simulink model "casperdemo"  (Simulink 6.2)
settings: Solver=ode45  StartTime=0.0  StopTime=16384  RelTol=1e-3
libraries: xbsIndex_r3 x1645, casper_library x163, testbench_lib x15, xps_library x1
(part 1 of 12)
settings Model: LastModifiedBy=Glenn
settings DebuggingCC: SolverPrmCheckMsg=warning

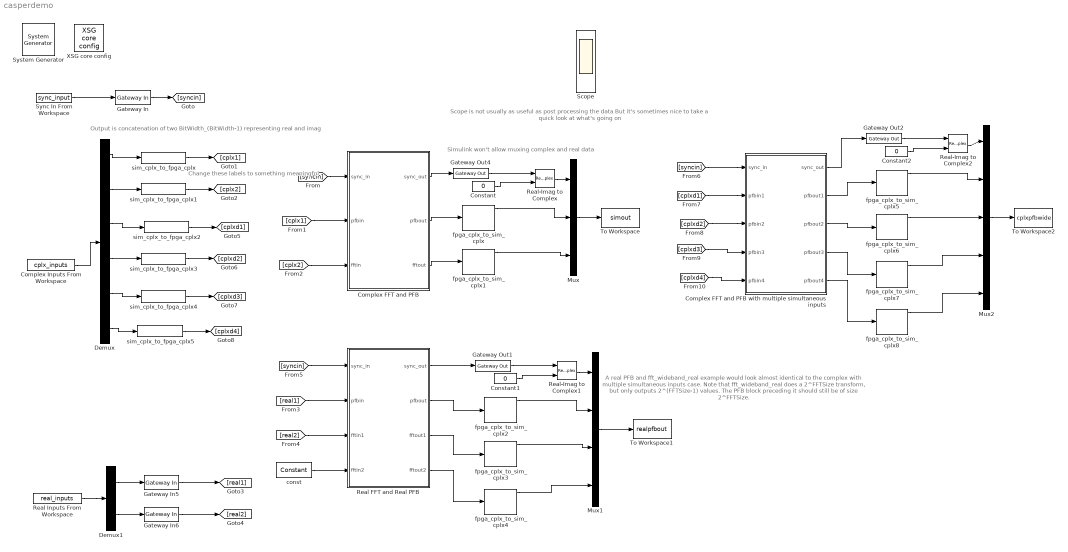
== system casperdemo ==
  note: Output is concatenation of two BitWidth_(BitWidth-1)
      | representing real and imag
  note: Change these labels to
      | something meaningful
  note: Simulink won't allow muxing
      | complex and real data
  note: Scope is not usually as useful as post processing the data
      | But it's sometimes nice to take a quick look at what's going on
  note: A real PFB and fft_wideband_real example would
      | look almost identical to the complex with multiple simultaneous
      | inputs case. Note that fft_wideband_real does a 2^FFTSize
      | transform, but only outputs 2^(FFTSize-1) values.
      | The PFB block preceding it should still be of size 2^FFTSize.
  " System Generator" : xbsIndex_r3/ System Generator  Tag=genX  xilinxfamily=Virtex2  part=xc2v1000  speed=-4  package=bg575  synthesis_tool=XST  directory=./netlist  testbench=off  simulink_period=1  sysclk_period=100  incr_netlist=off  trim_vbits=Everywhere in SubSystem  dbl_ovrd=According to Block Masks  core_generation=According to Block Masks  run_coregen=off  deprecated_control=off  eval_field=0
      settings: AttributesFormatString=System\nGenerator
  Complex FFT and PFB : Subsystem
  Complex FFT and PFB with multiple simultaneous inputs : Subsystem
  Complex Inputs From Workspace : FromWorkspace  VariableName=cplx_inputs  SampleTime=1  Interpolate=off  OutputAfterFinalValue=Setting to zero
  Constant : Constant  Value=0
  Constant1 : Constant  Value=0
  Constant2 : Constant  Value=0
  Demux : Demux  Outputs=6
  Demux1 : Demux  Outputs=2
  Gateway In : xbsIndex_r3/Gateway In  arith_type=Boolean  n_bits=8  bin_pt=6  quantization=Truncate  overflow=Wrap  period=1  timing_constraint=None  locs_specified=off  LOCs={}  needs_fixed_name=off  dbl_ovrd=off  show_param=off
      settings: xl_area=[0, 0, 0, 0, 0, 0, 0]
  Gateway In5 : xbsIndex_r3/Gateway In  arith_type="Signed  (2's comp)"  n_bits=8  bin_pt=7  quantization=Truncate  overflow=Wrap  period=1  timing_constraint=None  locs_specified=off  LOCs={}  needs_fixed_name=off  dbl_ovrd=off  show_param=off
      settings: xl_area=[0, 0, 0, 0, 0, 0, 0]
  Gateway In6 : xbsIndex_r3/Gateway In  arith_type="Signed  (2's comp)"  n_bits=18  bin_pt=17  quantization=Truncate  overflow=Wrap  period=1  timing_constraint=None  locs_specified=off  LOCs={}  needs_fixed_name=off  dbl_ovrd=off  show_param=off
      settings: xl_area=[0, 0, 0, 0, 0, 0, 0]
  Gateway Out1 : xbsIndex_r3/Gateway Out  output_type=Double  nbits=8  bin_pt=6  arith_type=Boolean  quantization=Truncate  overflow=Wrap  hdl_port=on  timing_constraint=None  locs_specified=off  LOCs={}  needs_fixed_name=off  show_param=off
      settings: xl_area=[0, 0, 0, 0, 0, 0, 0]
  Gateway Out2 : xbsIndex_r3/Gateway Out  output_type=Double  nbits=8  bin_pt=6  arith_type=Boolean  quantization=Truncate  overflow=Wrap  hdl_port=on  timing_constraint=None  locs_specified=off  LOCs={}  needs_fixed_name=off  show_param=off
      settings: xl_area=[0, 0, 0, 0, 0, 0, 0]
  Gateway Out4 : xbsIndex_r3/Gateway Out  output_type=Double  nbits=8  bin_pt=6  arith_type=Boolean  quantization=Truncate  overflow=Wrap  hdl_port=on  timing_constraint=None  locs_specified=off  LOCs={}  needs_fixed_name=off  show_param=off
      settings: xl_area=[0, 0, 0, 0, 0, 0, 0]
  Mux : Mux  Inputs=3
  Mux1 : Mux
  Mux2 : Mux  Inputs=5
  Real FFT and Real PFB : Subsystem
  Real Inputs From Workspace : FromWorkspace  VariableName=real_inputs  SampleTime=1  Interpolate=off  OutputAfterFinalValue=Setting to zero
  Real-Imag to Complex : RealImagToComplex
  Real-Imag to Complex1 : RealImagToComplex
  Real-Imag to Complex2 : RealImagToComplex
  Scope : Scope  NumInputPorts=4
      settings: YMin=-1~-0.5~-0.5~-1  YMax=1~0.5~0.5~1
  Sync In From Workspace : FromWorkspace  VariableName=sync_input  SampleTime=1  Interpolate=off  OutputAfterFinalValue=Setting to zero
  To Workspace : ToWorkspace  VariableName=simout  SampleTime=-1  SaveFormat=Structure
  To Workspace1 : ToWorkspace  VariableName=realpfbout  SampleTime=-1  SaveFormat=Structure
  To Workspace2 : ToWorkspace  VariableName=cplxpfbwide  SampleTime=-1  SaveFormat=Structure
  XSG core config : xps_library/XSG core config  Tag=xps:xsg  hw_sys=iBOB  ibob_linux=off  clk_src=sys_clk  gpio_clk_io_group=iBOB:sma  gpio_clk_bit_index=0  clk_rate=100  sample_period=1  synthesis_tool=XST  mpc_type=powerpc405
  const : xbsIndex_r3/Constant  const=.1  equ=P=C  arith_type="Signed  (2's comp)"  n_bits=18  bin_pt=17  opselect=C  inp2=PCIN>>17  opr=+  inp1=P  carry=CIN  iostate=0  explicit_period=on  period=1  dbl_ovrd=off
  fpga_cplx_to_sim_cplx{,1..8} (9 alike) : testbench_lib/fpga_cplx_to_sim_cplx  width=18
      settings: AttributesFormatString=18_17 bit
  sim_cplx_to_fpga_cplx{,2..5} (5 alike) : testbench_lib/sim_cplx_to_fpga_cplx  width=8
      settings: AttributesFormatString=8_7 bit
  sim_cplx_to_fpga_cplx1 : testbench_lib/sim_cplx_to_fpga_cplx  width=18
      settings: AttributesFormatString=18_17 bit
  wires:
  Sync In From Workspace/1 -> Gateway In/1
  Complex Inputs From Workspace/1 -> Demux/1
  Demux/1 -> sim_cplx_to_fpga_cplx/1
  Demux/2 -> sim_cplx_to_fpga_cplx1/1
  Real Inputs From Workspace/1 -> Demux1/1
  Demux1/1 -> Gateway In5/1
  Demux1/2 -> Gateway In6/1
  Gateway In/1 -> [syncin]
  sim_cplx_to_fpga_cplx/1 -> [cplx1]
  sim_cplx_to_fpga_cplx1/1 -> [cplx2]
  Gateway In5/1 -> [real1]
  Gateway In6/1 -> [real2]
  [syncin] -> Complex FFT and PFB/1(sync_in)
  [cplx1] -> Complex FFT and PFB/2(pfbin)
  Complex FFT and PFB/1(sync_out) -> Gateway Out4/1
  Complex FFT and PFB/2(pfbout) -> fpga_cplx_to_sim_cplx/1
  Complex FFT and PFB/3(fftout) -> fpga_cplx_to_sim_cplx1/1
  Gateway Out4/1 -> Real-Imag to Complex/1
  Constant/1 -> Real-Imag to Complex/2
  Real-Imag to Complex/1 -> Mux/1
  fpga_cplx_to_sim_cplx/1 -> Mux/2
  fpga_cplx_to_sim_cplx1/1 -> Mux/3
  Mux/1 -> To Workspace/1
  [cplx2] -> Complex FFT and PFB/3(fftin)
  [syncin] -> Real FFT and Real PFB/1(sync_in)
  [real1] -> Real FFT and Real PFB/2(pfbin)
  [real2] -> Real FFT and Real PFB/3(fftin1)
  const/1 -> Real FFT and Real PFB/4(fftin2)
  Gateway Out1/1 -> Real-Imag to Complex1/1
  Constant1/1 -> Real-Imag to Complex1/2
  Real-Imag to Complex1/1 -> Mux1/1
  fpga_cplx_to_sim_cplx2/1 -> Mux1/2
  fpga_cplx_to_sim_cplx3/1 -> Mux1/3
  Mux1/1 -> To Workspace1/1
  Real FFT and Real PFB/1(sync_out) -> Gateway Out1/1
  Real FFT and Real PFB/2(pfbout) -> fpga_cplx_to_sim_cplx2/1
  Real FFT and Real PFB/3(fftout1) -> fpga_cplx_to_sim_cplx3/1
  Real FFT and Real PFB/4(fftout2) -> fpga_cplx_to_sim_cplx4/1
  fpga_cplx_to_sim_cplx4/1 -> Mux1/4
  Demux/3 -> sim_cplx_to_fpga_cplx2/1
  Demux/4 -> sim_cplx_to_fpga_cplx3/1
  Demux/5 -> sim_cplx_to_fpga_cplx4/1
  Demux/6 -> sim_cplx_to_fpga_cplx5/1
  sim_cplx_to_fpga_cplx2/1 -> [cplxd1]
  sim_cplx_to_fpga_cplx3/1 -> [cplxd2]
  sim_cplx_to_fpga_cplx4/1 -> [cplxd3]
  sim_cplx_to_fpga_cplx5/1 -> [cplxd4]
  [syncin] -> Complex FFT and PFB with multiple simultaneous inputs/1(sync_in)
  [cplxd1] -> Complex FFT and PFB with multiple simultaneous inputs/2(pfbin1)
  [cplxd2] -> Complex FFT and PFB with multiple simultaneous inputs/3(pfbin2)
  [cplxd3] -> Complex FFT and PFB with multiple simultaneous inputs/4(pfbin3)
  [cplxd4] -> Complex FFT and PFB with multiple simultaneous inputs/5(pfbin4)
  Gateway Out2/1 -> Real-Imag to Complex2/1
  Constant2/1 -> Real-Imag to Complex2/2
  Real-Imag to Complex2/1 -> Mux2/1
  fpga_cplx_to_sim_cplx5/1 -> Mux2/2
  fpga_cplx_to_sim_cplx6/1 -> Mux2/3
  Mux2/1 -> To Workspace2/1
  fpga_cplx_to_sim_cplx7/1 -> Mux2/4
  fpga_cplx_to_sim_cplx8/1 -> Mux2/5
  Complex FFT and PFB with multiple simultaneous inputs/1(sync_out) -> Gateway Out2/1
  Complex FFT and PFB with multiple simultaneous inputs/2(pfbout1) -> fpga_cplx_to_sim_cplx5/1
  Complex FFT and PFB with multiple simultaneous inputs/3(pfbout2) -> fpga_cplx_to_sim_cplx6/1
  Complex FFT and PFB with multiple simultaneous inputs/4(pfbout3) -> fpga_cplx_to_sim_cplx7/1
  Complex FFT and PFB with multiple simultaneous inputs/5(pfbout4) -> fpga_cplx_to_sim_cplx8/1

== system casperdemo/Complex FFT and PFB ==
  note: With "Number of Simultaneous Inputs" = 2^0,
      | each input represents an independant data stream
      | processed simultaneously by the biplex structure.
      | Each segment of the input time series
      |  of length 2^FFTSize is transformed and
      | output as 2^FFTSize frequency points.
  sync_in : Inport  Port=1  LatchInput=off
  pfbin : Inport  Port=2  LatchInput=off
  fftin : Inport  Port=3  LatchInput=off
  fft : Subsystem  AncestorBlock=casper_library/FFTs/fft  mask(fft){FFTSize=4, BitWidth=18, n_inputs=0, quantization=Truncate, overflow=Wrap, add_latency=2, mult_latency=3, bram_latency=2}
      mask prompts: FFTSize "Size of FFT: (2^?)"; BitWidth "Bit Width"; n_inputs "Number of Simultaneous Inputs: (2^?)"; quantization "Quantization Behavior"; overflow "Overflow Behavior"; add_latency "Add Latency"; mult_latency "Mult Latency"; bram_latency "BRAM Latency"
      mask init:
      | fft_init(gcb,...
      |     'FFTSize', FFTSize,...
      |     'BitWidth', BitWidth,...
      |     'n_inputs', n_inputs,...
      |     'quantization', quantization,...
      |     'overflow', overflow,...
      |     'add_latency', add_latency,...
      |     'mult_latency', mult_latency,...
      |     'bram_latency', bram_latency);
      settings: AttributesFormatString=FFTSize=4, n_inputs=0
      mask StyleString: edit,edit,edit,popup(Truncate|Round  (unbiased: +/- Inf)|Round  (unbiased: Even Values)),popup(Wrap|Saturate|Error),edit,edit,edit
  pfb_fir : Subsystem  AncestorBlock=casper_library/PFBs/pfb_fir  mask(pfb_fir){PFBSize=4, TotalTaps=4, WindowType=hamming, n_inputs=0, MakeBiplex=1, BitWidthIn=8, BitWidthOut=18, CoeffBitWidth=8, CoeffDistMem=1, add_latency=1, mult_latency=2, bram_latency=2, quantization=Truncate, fwidth=1}
      mask prompts: PFBSize "Size of PFB: (2^? pnts)"; TotalTaps "Total Number of Taps:"; WindowType "Windowing Function:"; n_inputs "Number of Simultaneous Inputs: (2^?)"; MakeBiplex "Make Biplex"; BitWidthIn "Input Bitwidth:"; BitWidthOut "Output Bitwidth:"; CoeffBitWidth "Coefficient Bitwidth:"; CoeffDistMem "Use Distributed Memory for Coeffs"; add_latency "Add Latency"; mult_latency "Mult Latency"; bram_latency "BRAM Latency"; quantization "Quantization Behavior"; fwidth "Bin Width Scaling (normal=1)"
      mask init:
      | pfb_fir_init(gcb, ...
      |     'PFBSize', PFBSize, ...
      |     'TotalTaps', TotalTaps, ...
      |     'WindowType', WindowType, ...
      |     'n_inputs', n_inputs, ...
      |     'MakeBiplex', MakeBiplex, ...
      |     'BitWidthIn', BitWidthIn, ...
      |     'BitWidthOut', BitWidthOut, ...
      |     'CoeffBitWidth', CoeffBitWidth, ...
      |     'CoeffDistMem', CoeffDistMem, ...
      |     'add_latency', add_latency, ...
      |     'mult_latency', mult_latency, ...
      |     'bram_latency', bram_latency, ...
      |     'quantization', quantization, ...
      |     'fwidth', fwidth);
      settings: AttributesFormatString=taps=4, add_latency=1
      mask StyleString: edit,edit,popup(bartlett|barthannwin|blackman|blackmanharris|bohamwin|chebwin|flattopwin|gausswin|hamming|hann|kaiser|nuttallwin|parzenwin|rectwin|tukeywin|triang),edit,edit,edit,edit,edit,edit,edit,edit,edit,popup(Truncate|Round  (unbiased: +/- Inf)|Round  (unbiased: Even Values)),edit
  shift : xbsIndex_r3/Constant  const=-1  equ=P=C  arith_type="Signed  (2's comp)"  n_bits=32  bin_pt=0  opselect=C  inp2=PCIN>>17  opr=+  inp1=P  carry=CIN  iostate=0  explicit_period=on  period=1  dbl_ovrd=off
  sync_out : Outport
  pfbout : Outport  Port=2
  fftout : Outport  Port=3
  wires:
  sync_in/1 -> pfb_fir/1(sync)
  fft/1(sync_out) -> sync_out/1
  shift/1 -> fft/2(shift)
  fft/2(out0) -> pfbout/1
  fft/3(out1) -> fftout/1
  pfb_fir/1(sync_out) -> fft/1(sync)
  pfb_fir/2(pol1_out1) -> fft/3(pol0)
  pfbin/1 -> pfb_fir/2(pol1_in1), pfb_fir/3(pol2_in1)
  fftin/1 -> fft/4(pol1)

== system casperdemo/Complex FFT and PFB with multiple simultaneous inputs ==
  note: With "Number of Simultaneous Inputs" = 2^2,
      | the four inputs represent successive time samples
      | of the overall timeseries. They should be thought of in
      | blocks, for example as (x0,x1,x2,x3) come in on one clock
      | then (x4,x5,x6,x7) on the next clock. The outputs come out in
      | the same fashion. Thus if FFTSize=5, with 4 inputs at a time,
      | we get a full spectrum every 32/4 = 8 clocks.
  note: This could be hooked to a set of four
      | real/imag to complex blocks, with
      | the real ports driven by the I ADC inputs
      | and the imag ports driven by the Q ADC inputs
  sync_in : Inport  Port=1  LatchInput=off
  pfbin1 : Inport  Port=2  LatchInput=off
  pfbin2 : Inport  Port=3  LatchInput=off
  pfbin3 : Inport  Port=4  LatchInput=off
  pfbin4 : Inport  Port=5  LatchInput=off
  fft : Subsystem  AncestorBlock=casper_library/FFTs/fft  mask(fft){FFTSize=5, BitWidth=18, n_inputs=2, quantization=Truncate, overflow=Wrap, add_latency=2, mult_latency=3, bram_latency=2}
      mask prompts: FFTSize "Size of FFT: (2^?)"; BitWidth "Bit Width"; n_inputs "Number of Simultaneous Inputs: (2^?)"; quantization "Quantization Behavior"; overflow "Overflow Behavior"; add_latency "Add Latency"; mult_latency "Mult Latency"; bram_latency "BRAM Latency"
      mask init: same as casperdemo/Complex FFT and PFB/fft
      settings: AttributesFormatString=FFTSize=5, n_inputs=2
      mask StyleString: edit,edit,edit,popup(Truncate|Round  (unbiased: +/- Inf)|Round  (unbiased: Even Values)),popup(Wrap|Saturate|Error),edit,edit,edit
  pfb_fir : Subsystem  AncestorBlock=casper_library/PFBs/pfb_fir  mask(pfb_fir){PFBSize=5, TotalTaps=4, WindowType=hamming, n_inputs=2, MakeBiplex=0, BitWidthIn=8, BitWidthOut=18, CoeffBitWidth=8, CoeffDistMem=1, add_latency=1, mult_latency=2, bram_latency=2, quantization=Truncate, fwidth=1}
      mask prompts: PFBSize "Size of PFB: (2^? pnts)"; TotalTaps "Total Number of Taps:"; WindowType "Windowing Function:"; n_inputs "Number of Simultaneous Inputs: (2^?)"; MakeBiplex "Make Biplex"; BitWidthIn "Input Bitwidth:"; BitWidthOut "Output Bitwidth:"; CoeffBitWidth "Coefficient Bitwidth:"; CoeffDistMem "Use Distributed Memory for Coeffs"; add_latency "Add Latency"; mult_latency "Mult Latency"; bram_latency "BRAM Latency"; quantization "Quantization Behavior"; fwidth "Bin Width Scaling (normal=1)"
      mask init: same as casperdemo/Complex FFT and PFB/pfb_fir
      settings: AttributesFormatString=taps=4, add_latency=1
      mask StyleString: edit,edit,popup(bartlett|barthannwin|blackman|blackmanharris|bohamwin|chebwin|flattopwin|gausswin|hamming|hann|kaiser|nuttallwin|parzenwin|rectwin|tukeywin|triang),edit,edit,edit,edit,edit,edit,edit,edit,edit,popup(Truncate|Round  (unbiased: +/- Inf)|Round  (unbiased: Even Values)),edit
  shift : xbsIndex_r3/Constant  const=-1  equ=P=C  arith_type="Signed  (2's comp)"  n_bits=32  bin_pt=0  opselect=C  inp2=PCIN>>17  opr=+  inp1=P  carry=CIN  iostate=0  explicit_period=on  period=1  dbl_ovrd=off
  sync_out : Outport
  pfbout1 : Outport  Port=2
  pfbout2 : Outport  Port=3
  pfbout3 : Outport  Port=4
  pfbout4 : Outport  Port=5
  wires:
  pfbin1/1 -> pfb_fir/2(pol1_in1)
  pfb_fir/1(sync_out) -> fft/1(sync)
  shift/1 -> fft/2(shift)
  fft/1(sync_out) -> sync_out/1
  sync_in/1 -> pfb_fir/1(sync)
  pfb_fir/2(pol1_out1) -> fft/3(in0)
  pfb_fir/3(pol1_out2) -> fft/4(in1)
  pfb_fir/4(pol1_out3) -> fft/5(in2)
  pfb_fir/5(pol1_out4) -> fft/6(in3)
  pfbin2/1 -> pfb_fir/3(pol1_in2)
  pfbin3/1 -> pfb_fir/4(pol1_in3)
  pfbin4/1 -> pfb_fir/5(pol1_in4)
  fft/2(out0) -> pfbout1/1
  fft/3(out1) -> pfbout2/1
  fft/4(out2) -> pfbout3/1
  fft/5(out3) -> pfbout4/1

== system casperdemo/Real FFT and Real PFB ==
  note: Each input represents an independant data stream
      | Each segment of the input time series
      |  of length 2^FFTSize is transformed and
      | output as 2^FFTSize frequency points.
      | Negative frequencies included.
  sync_in : Inport  Port=1  LatchInput=off
  pfbin : Inport  Port=2  LatchInput=off
  fftin1 : Inport  Port=3  LatchInput=off
  fftin2 : Inport  Port=4  LatchInput=off
  fft_biplex_real_4x : Subsystem  AncestorBlock=casper_library/FFTs/fft_biplex_real_4x  mask(fft_biplex_real_4x){FFTSize=4, BitWidth=18, quantization=Truncate, overflow=Wrap, add_latency=2, mult_latency=3, bram_latency=2}
      mask prompts: FFTSize "Size of FFT: (2^? pnts)"; BitWidth "Bitwidth: (Max Efficiency at 18 bits)"; quantization "Quantization Behavior"; overflow "Overflow Behavior"; add_latency "Add Latency"; mult_latency "Mult Latency"; bram_latency "BRAM Latency"
      mask init:
      | fft_biplex_real_4x_init(gcb,...
      |     'FFTSize', FFTSize,...
      |     'BitWidth', BitWidth,...
      |     'quantization', quantization,...
      |     'overflow', overflow,...
      |     'add_latency', add_latency,...
      |     'mult_latency', mult_latency,...
      |     'bram_latency', bram_latency);
      settings: AttributesFormatString=FFTSize=4, BitWidth=18
      mask StyleString: edit,edit,popup(Truncate|Round  (unbiased: +/- Inf)|Round  (unbiased: Even Values)),popup(Wrap|Saturate|Error),edit,edit,edit
  pfb_fir_real : Subsystem  AncestorBlock=casper_library/PFBs/pfb_fir_real  mask(pfb_fir_real){PFBSize=4, TotalTaps=4, WindowType=hamming, n_inputs=0, MakeBiplex=0, BitWidthIn=8, BitWidthOut=18, CoeffBitWidth=8, CoeffDistMem=1, add_latency=1, mult_latency=2, bram_latency=2, quantization=Truncate, fwidth=1}
      mask prompts: PFBSize "Size of PFB: (2^? pnts)"; TotalTaps "Total Number of Taps:"; WindowType "Windowing Function:"; n_inputs "Number of Simultaneous Inputs: (2^?)"; MakeBiplex "Make Biplex"; BitWidthIn "Input Bitwidth:"; BitWidthOut "Output Bitwidth:"; CoeffBitWidth "Coefficient Bitwidth:"; CoeffDistMem "Use Distributed Memory for Coeffs"; add_latency "Add Latency"; mult_latency "Mult Latency"; bram_latency "BRAM Latency"; quantization "Quantization Behavior"; fwidth "Bin Width Scaling (normal=1)"
      mask init:
      | pfb_fir_real_init(gcb,...
      |     'PFBSize', PFBSize,...
      |     'TotalTaps', TotalTaps,...
      |     'WindowType', WindowType,...
      |     'n_inputs', n_inputs,...
      |     'MakeBiplex', MakeBiplex,...
      |     'BitWidthIn', BitWidthIn,...
      |     'BitWidthOut', BitWidthOut,...
      |     'CoeffBitWidth', CoeffBitWidth,...
      |     'CoeffDistMem', CoeffDistMem,...
      |     'add_latency', add_latency,...
      |     'mult_latency', mult_latency,...
      |     'bram_latency', bram_latency,...
      |     'quantization', quantization,...
      |     'fwidth', fwidth);
      settings: AttributesFormatString=taps=4, add_latency=1
      mask StyleString: edit,edit,popup(bartlett|barthannwin|blackman|blackmanharris|bohamwin|chebwin|flattopwin|gausswin|hamming|hann|kaiser|nuttallwin|parzenwin|rectwin|tukeywin|triang),edit,edit,edit,edit,edit,edit,edit,edit,edit,popup(Truncate|Round  (unbiased: +/- Inf)|Round  (unbiased: Even Values)),edit
  shift : xbsIndex_r3/Constant  const=-1  equ=P=C  arith_type="Signed  (2's comp)"  n_bits=32  bin_pt=0  opselect=C  inp2=PCIN>>17  opr=+  inp1=P  carry=CIN  iostate=0  explicit_period=on  period=1  dbl_ovrd=off
  sync_out : Outport
  pfbout : Outport  Port=2
  fftout1 : Outport  Port=3
  fftout2 : Outport  Port=4
  wires:
  pfbin/1 -> pfb_fir_real/2(pol1_in1)
  sync_in/1 -> pfb_fir_real/1(sync)
  fftin2/1 -> fft_biplex_real_4x/3(pol3), fft_biplex_real_4x/4(pol4)
  shift/1 -> fft_biplex_real_4x/6(shift)
  fft_biplex_real_4x/6(sync_out) -> sync_out/1
  fft_biplex_real_4x/1(pol1_out) -> pfbout/1
  fft_biplex_real_4x/2(pol2_out) -> fftout1/1
  fft_biplex_real_4x/3(pol3_out) -> fftout2/1
  pfb_fir_real/2(pol1_out1) -> fft_biplex_real_4x/1(pol1)
  fftin1/1 -> fft_biplex_real_4x/2(pol2)
  pfb_fir_real/1(sync_out) -> fft_biplex_real_4x/5(sync)

== system casperdemo/Complex FFT and PFB/fft ==
  sync : Inport  Port=1  LatchInput=off
  shift : Inport  Port=2  LatchInput=off
  pol0 : Inport  Port=3  LatchInput=off
  pol1 : Inport  Port=4  LatchInput=off
  fft_biplex0 : Subsystem  AncestorBlock=casper_library/FFTs/fft_biplex  mask(fft_biplex){FFTSize=4, BitWidth=18, quantization=Truncate, overflow=Wrap, add_latency=2, mult_latency=3, bram_latency=2}
      mask prompts: FFTSize "Size of FFT: (2^? pnts)"; BitWidth "Bitwidth: (Max Efficiency at 18 bits)"; quantization "Quantization Behavior"; overflow "Overflow Behavior"; add_latency "Add Latency"; mult_latency "Mult Latency"; bram_latency "BRAM Latency"
      mask init:
      | fft_biplex_init(gcb,...
      |     'FFTSize', FFTSize,...
      |     'BitWidth', BitWidth,...
      |     'quantization', quantization,...
      |     'overflow', overflow,...
      |     'add_latency', add_latency,...
      |     'mult_latency', mult_latency,...
      |     'bram_latency', bram_latency);
      settings: AttributesFormatString=FFTSize=4, BitWidth=18
      mask StyleString: edit,edit,popup(Truncate|Round  (unbiased: +/- Inf)|Round  (unbiased: Even Values)),popup(Wrap|Saturate|Error),edit,edit,edit
  sync_out : Outport
  out0 : Outport  Port=2
  out1 : Outport  Port=3
  wires:
  pol0/1 -> fft_biplex0/1(pol1)
  pol1/1 -> fft_biplex0/2(pol2)
  shift/1 -> fft_biplex0/4(shift)
  sync/1 -> fft_biplex0/3(sync)
  fft_biplex0/1(pol1_out) -> out0/1
  fft_biplex0/2(pol2_out) -> out1/1
  fft_biplex0/4(sync_out) -> sync_out/1

== system casperdemo/Complex FFT and PFB/pfb_fir ==
  sync : Inport  Port=1  LatchInput=off
  pol1_in1 : Inport  Port=2  LatchInput=off
  pol2_in1 : Inport  Port=3  LatchInput=off
  pol1_in1_first_tap : Subsystem  AncestorBlock=casper_library/PFBs/first_tap  mask(first_tap){nput=0, PFBSize=4, CoeffBitWidth=8, TotalTaps=4, BitWidthIn=8, CoeffDistMem=1, WindowType=hamming, mult_latency=2, bram_latency=2, n_inputs=0, fwidth=1}
      mask prompts: nput "This is input number:"; PFBSize "Size of PFB: (2^? pnts)"; CoeffBitWidth "Bitwidth of Coefficients:"; TotalTaps "Total Number of Taps:"; BitWidthIn "Input Bitwidth:"; CoeffDistMem "Implement Coeff Gen in Distributed Memory:"; WindowType "Windowing Function:"; mult_latency "Mult Latency"; bram_latency "BRAM Latency"; n_inputs "Number of Simultaneous Inputs: (2^?)"; fwidth "Bit Width (normal=1)"
      mask init:
      | first_tap_init(gcb,...
      |     'nput', nput,...
      |     'PFBSize', PFBSize,...
      |     'CoeffBitWidth', CoeffBitWidth,...
      |     'TotalTaps', TotalTaps,...
      |     'BitWidthIn', BitWidthIn,...
      |     'CoeffDistMem', CoeffDistMem,...
      |     'WindowType', WindowType,...
      |     'mult_latency', mult_latency,...
      |     'bram_latency', bram_latency,...
      |     'n_inputs', n_inputs,...
      |     'fwidth', fwidth);
      settings: AttributesFormatString=input=0, taps=4
      mask StyleString: edit,edit,edit,edit,edit,edit,popup(bartlett|barthannwin|blackman|blackmanharris|bohamwin|chebwin|flattopwin|gausswin|hamming|hann|kaiser|nuttallwin|parzenwin|rectwin|tukeywin|triang),edit,edit,edit,edit
  pol1_in1_last_tap : Subsystem  AncestorBlock=casper_library/PFBs/last_tap  mask(last_tap){TotalTaps=4, BitWidthIn=8, BitWidthOut=18, CoeffBitWidth=8, add_latency=1, mult_latency=2, quantization=Truncate}
      mask prompts: TotalTaps "Total Number of Taps:"; BitWidthIn "Input Bitwidth:"; BitWidthOut "Output Bitwidth:"; CoeffBitWidth "Coeff Bitwidth:"; add_latency "Add Latency"; mult_latency "Mult Latency"; quantization "Quantization Behavior"
      mask init:
      | last_tap_init(gcb,...
      |     'TotalTaps', TotalTaps,...
      |     'BitWidthIn', BitWidthIn,...
      |     'BitWidthOut', BitWidthOut,...
      |     'CoeffBitWidth', CoeffBitWidth,...
      |     'add_latency', add_latency,...
      |     'mult_latency', mult_latency,...
      |     'quantization', quantization);
      settings: AttributesFormatString=taps=4
      mask StyleString: edit,edit,edit,edit,edit,edit,popup(Truncate|Round  (unbiased: +/- Inf)|Round  (unbiased: Even Values))
  pol1_in1_tap2 : casper_library/PFBs/tap
      link override delay/delay_bram/Constant2: equ=P=C
      link override sync_delay/Constant: equ=P=C
      link override sync_delay/Constant1: equ=P=C
      link override sync_delay/Constant2: equ=P=C
      link override sync_delay/Constant3: equ=P=C
  pol1_in1_tap3 : casper_library/PFBs/tap
      link override delay/delay_bram/Constant2: equ=P=C
      link override sync_delay/Constant: equ=P=C
      link override sync_delay/Constant1: equ=P=C
      link override sync_delay/Constant2: equ=P=C
      link override sync_delay/Constant3: equ=P=C
  pol2_in1_first_tap : Subsystem  AncestorBlock=casper_library/PFBs/first_tap  mask(first_tap){nput=0, PFBSize=4, CoeffBitWidth=8, TotalTaps=4, BitWidthIn=8, CoeffDistMem=1, WindowType=hamming, mult_latency=2, bram_latency=2, n_inputs=0, fwidth=1}
      mask prompts: nput "This is input number:"; PFBSize "Size of PFB: (2^? pnts)"; CoeffBitWidth "Bitwidth of Coefficients:"; TotalTaps "Total Number of Taps:"; BitWidthIn "Input Bitwidth:"; CoeffDistMem "Implement Coeff Gen in Distributed Memory:"; WindowType "Windowing Function:"; mult_latency "Mult Latency"; bram_latency "BRAM Latency"; n_inputs "Number of Simultaneous Inputs: (2^?)"; fwidth "Bit Width (normal=1)"
      mask init: same as casperdemo/Complex FFT and PFB/pfb_fir/pol1_in1_first_tap
      settings: AttributesFormatString=input=0, taps=4
      mask StyleString: edit,edit,edit,edit,edit,edit,popup(bartlett|barthannwin|blackman|blackmanharris|bohamwin|chebwin|flattopwin|gausswin|hamming|hann|kaiser|nuttallwin|parzenwin|rectwin|tukeywin|triang),edit,edit,edit,edit
  pol2_in1_last_tap : Subsystem  AncestorBlock=casper_library/PFBs/last_tap  mask(last_tap){TotalTaps=4, BitWidthIn=8, BitWidthOut=18, CoeffBitWidth=8, add_latency=1, mult_latency=2, quantization=Truncate}
      mask prompts: TotalTaps "Total Number of Taps:"; BitWidthIn "Input Bitwidth:"; BitWidthOut "Output Bitwidth:"; CoeffBitWidth "Coeff Bitwidth:"; add_latency "Add Latency"; mult_latency "Mult Latency"; quantization "Quantization Behavior"
      mask init: same as casperdemo/Complex FFT and PFB/pfb_fir/pol1_in1_last_tap
      settings: AttributesFormatString=taps=4
      mask StyleString: edit,edit,edit,edit,edit,edit,popup(Truncate|Round  (unbiased: +/- Inf)|Round  (unbiased: Even Values))
  pol2_in1_tap2 : casper_library/PFBs/tap
      link override delay/delay_bram/Constant2: equ=P=C
      link override sync_delay/Constant: equ=P=C
      link override sync_delay/Constant1: equ=P=C
      link override sync_delay/Constant2: equ=P=C
      link override sync_delay/Constant3: equ=P=C
  pol2_in1_tap3 : casper_library/PFBs/tap
      link override delay/delay_bram/Constant2: equ=P=C
      link override sync_delay/Constant: equ=P=C
      link override sync_delay/Constant1: equ=P=C
      link override sync_delay/Constant2: equ=P=C
      link override sync_delay/Constant3: equ=P=C
  sync_out : Outport
  pol1_out1 : Outport  Port=2
  pol2_out1 : Outport  Port=3
  wires:
  pol1_in1/1 -> pol1_in1_first_tap/1(din)
  sync/1 -> pol1_in1_first_tap/2(sync), pol2_in1_first_tap/2(sync)
  pol1_in1_first_tap/1(dout) -> pol1_in1_tap2/1
  pol1_in1_first_tap/2(sync_out) -> pol1_in1_tap2/2
  pol1_in1_first_tap/3(coeff_out) -> pol1_in1_tap2/3
  pol1_in1_first_tap/4(taps_out) -> pol1_in1_tap2/4
  pol1_in1_tap2/1 -> pol1_in1_tap3/1
  pol1_in1_tap2/2 -> pol1_in1_tap3/2
  pol1_in1_tap2/3 -> pol1_in1_tap3/3
  pol1_in1_tap2/4 -> pol1_in1_tap3/4
  pol1_in1_tap3/1 -> pol1_in1_last_tap/1(din)
  pol1_in1_tap3/2 -> pol1_in1_last_tap/2(sync)
  pol1_in1_tap3/3 -> pol1_in1_last_tap/3(coeff)
  pol1_in1_tap3/4 -> pol1_in1_last_tap/4(taps)
  pol1_in1_last_tap/1(dout) -> pol1_out1/1
  pol1_in1_last_tap/2(sync_out) -> sync_out/1
  pol2_in1/1 -> pol2_in1_first_tap/1(din)
  pol2_in1_first_tap/1(dout) -> pol2_in1_tap2/1
  pol2_in1_first_tap/2(sync_out) -> pol2_in1_tap2/2
  pol2_in1_first_tap/3(coeff_out) -> pol2_in1_tap2/3
  pol2_in1_first_tap/4(taps_out) -> pol2_in1_tap2/4
  pol2_in1_tap2/1 -> pol2_in1_tap3/1
  pol2_in1_tap2/2 -> pol2_in1_tap3/2
  pol2_in1_tap2/3 -> pol2_in1_tap3/3
  pol2_in1_tap2/4 -> pol2_in1_tap3/4
  pol2_in1_tap3/1 -> pol2_in1_last_tap/1(din)
  pol2_in1_tap3/2 -> pol2_in1_last_tap/2(sync)
  pol2_in1_tap3/3 -> pol2_in1_last_tap/3(coeff)
  pol2_in1_tap3/4 -> pol2_in1_last_tap/4(taps)
  pol2_in1_last_tap/1(dout) -> pol2_out1/1

== system casperdemo/Complex FFT and PFB with multiple simultaneous inputs/fft ==
  sync : Inport  Port=1  LatchInput=off
  shift : Inport  Port=2  LatchInput=off
  in0 : Inport  Port=3  LatchInput=off
  in1 : Inport  Port=4  LatchInput=off
  in2 : Inport  Port=5  LatchInput=off
  in3 : Inport  Port=6  LatchInput=off
  fft_biplex0 : Subsystem  AncestorBlock=casper_library/FFTs/fft_biplex  mask(fft_biplex){FFTSize=3, BitWidth=18, quantization=Truncate, overflow=Wrap, add_latency=2, mult_latency=3, bram_latency=2}
      mask prompts: FFTSize "Size of FFT: (2^? pnts)"; BitWidth "Bitwidth: (Max Efficiency at 18 bits)"; quantization "Quantization Behavior"; overflow "Overflow Behavior"; add_latency "Add Latency"; mult_latency "Mult Latency"; bram_latency "BRAM Latency"
      mask init: same as casperdemo/Complex FFT and PFB/fft/fft_biplex0
      settings: AttributesFormatString=FFTSize=3, BitWidth=18
      mask StyleString: edit,edit,popup(Truncate|Round  (unbiased: +/- Inf)|Round  (unbiased: Even Values)),popup(Wrap|Saturate|Error),edit,edit,edit
  fft_biplex1 : Subsystem  AncestorBlock=casper_library/FFTs/fft_biplex  mask(fft_biplex){FFTSize=3, BitWidth=18, quantization=Truncate, overflow=Wrap, add_latency=2, mult_latency=3, bram_latency=2}
      mask prompts: FFTSize "Size of FFT: (2^? pnts)"; BitWidth "Bitwidth: (Max Efficiency at 18 bits)"; quantization "Quantization Behavior"; overflow "Overflow Behavior"; add_latency "Add Latency"; mult_latency "Mult Latency"; bram_latency "BRAM Latency"
      mask init: same as casperdemo/Complex FFT and PFB/fft/fft_biplex0
      settings: AttributesFormatString=FFTSize=3, BitWidth=18
      mask StyleString: edit,edit,popup(Truncate|Round  (unbiased: +/- Inf)|Round  (unbiased: Even Values)),popup(Wrap|Saturate|Error),edit,edit,edit
  fft_direct : Subsystem  AncestorBlock=casper_library/FFTs/fft_direct  mask(fft_direct){FFTSize=2, BitWidth=18, add_latency=2, mult_latency=3, bram_latency=2, quantization=Truncate, overflow=Wrap, MapTail=1, LargerFFTSize=5, StartStage=4}
      mask prompts: FFTSize "Size of FFT: (2^?)"; BitWidth "Bit Width"; add_latency "Add Latency"; mult_latency "Mult Latency"; bram_latency "BRAM Latency"; quantization "Quantization Behavior"; overflow "Overflow Behavior"; MapTail "Map Tail of Larger FFT"; LargerFFTSize "Size of Larger FFT (2^?):"; StartStage "Start Stage of Map Tail:"
      mask init:
      | fft_direct_init(gcb,...
      |     'FFTSize', FFTSize,...
      |     'BitWidth', BitWidth,...
      |     'add_latency', add_latency,...
      |     'mult_latency', mult_latency,...
      |     'bram_latency', bram_latency,...
      |     'quantization', quantization,...
      |     'overflow', overflow,...
      |     'MapTail', MapTail,...
      |     'LargerFFTSize', LargerFFTSize,...
      |     'StartStage', StartStage);
      settings: AttributesFormatString=FFTSize=2
      mask StyleString: edit,edit,edit,edit,edit,popup(Truncate|Round  (unbiased: +/- Inf)|Round  (unbiased: Even Values)),popup(Wrap|Saturate|Error),edit,edit,edit
  fft_unscrambler : Subsystem  AncestorBlock=casper_library/FFTs/fft_unscrambler  mask(fft_unscrambler){FFTSize=5, n_inputs=2, bram_latency=2}
      mask prompts: FFTSize "Size of FFT: (2^?)"; n_inputs "Number of Simultaneous Inputs: (2^?)"; bram_latency "BRAM Latency"
      mask init:
      | fft_unscrambler_init(gcb,...
      |     'FFTSize',FFTSize,... 
      |     'n_inputs', n_inputs,...
      |     'bram_latency', bram_latency);
      settings: AttributesFormatString=FFTSize=5, n_inputs=2
  slice : xbsIndex_r3/Slice  mode=Lower Bit Location + Width  nbits=2  bit1=0  base1=MSB of Input  bit0=3  base0=LSB of Input  boolean_output=off  explicit_period=off  period=1  dbl_ovrd=off
  sync_out : Outport
  out0 : Outport  Port=2
  out1 : Outport  Port=3
  out2 : Outport  Port=4
  out3 : Outport  Port=5
  wires:
  in0/1 -> fft_biplex0/1(pol1)
  in1/1 -> fft_biplex0/2(pol2)
  shift/1 -> fft_biplex0/4(shift), fft_biplex1/4(shift), slice/1
  sync/1 -> fft_biplex0/3(sync), fft_biplex1/3(sync)
  in2/1 -> fft_biplex1/1(pol1)
  in3/1 -> fft_biplex1/2(pol2)
  slice/1 -> fft_direct/2(shift)
  fft_biplex0/4(sync_out) -> fft_direct/1(sync)
  fft_biplex0/1(pol1_out) -> fft_direct/3(in0)
  fft_biplex0/2(pol2_out) -> fft_direct/4(in1)
  fft_biplex1/1(pol1_out) -> fft_direct/5(in2)
  fft_biplex1/2(pol2_out) -> fft_direct/6(in3)
  fft_direct/1(sync_out) -> fft_unscrambler/1(sync)
  fft_unscrambler/1(sync_out) -> sync_out/1
  fft_direct/2(out0) -> fft_unscrambler/2(In1)
  fft_unscrambler/2(Out1) -> out0/1
  fft_direct/3(out1) -> fft_unscrambler/3(In2)
  fft_unscrambler/3(Out2) -> out1/1
  fft_direct/4(out2) -> fft_unscrambler/4(In3)
  fft_unscrambler/4(Out3) -> out2/1
  fft_direct/5(out3) -> fft_unscrambler/5(In4)
  fft_unscrambler/5(Out4) -> out3/1

== system casperdemo/Complex FFT and PFB with multiple simultaneous inputs/pfb_fir ==
  sync : Inport  Port=1  LatchInput=off
  pol1_in1 : Inport  Port=2  LatchInput=off
  pol1_in2 : Inport  Port=3  LatchInput=off
  pol1_in3 : Inport  Port=4  LatchInput=off
  pol1_in4 : Inport  Port=5  LatchInput=off
  pol1_in1_first_tap : Subsystem  AncestorBlock=casper_library/PFBs/first_tap  mask(first_tap){nput=0, PFBSize=5, CoeffBitWidth=8, TotalTaps=4, BitWidthIn=8, CoeffDistMem=1, WindowType=hamming, mult_latency=2, bram_latency=2, n_inputs=2, fwidth=1}
      mask prompts: nput "This is input number:"; PFBSize "Size of PFB: (2^? pnts)"; CoeffBitWidth "Bitwidth of Coefficients:"; TotalTaps "Total Number of Taps:"; BitWidthIn "Input Bitwidth:"; CoeffDistMem "Implement Coeff Gen in Distributed Memory:"; WindowType "Windowing Function:"; mult_latency "Mult Latency"; bram_latency "BRAM Latency"; n_inputs "Number of Simultaneous Inputs: (2^?)"; fwidth "Bit Width (normal=1)"
      mask init: same as casperdemo/Complex FFT and PFB/pfb_fir/pol1_in1_first_tap
      settings: AttributesFormatString=input=0, taps=4
      mask StyleString: edit,edit,edit,edit,edit,edit,popup(bartlett|barthannwin|blackman|blackmanharris|bohamwin|chebwin|flattopwin|gausswin|hamming|hann|kaiser|nuttallwin|parzenwin|rectwin|tukeywin|triang),edit,edit,edit,edit
  pol1_in1_last_tap : Subsystem  AncestorBlock=casper_library/PFBs/last_tap  mask(last_tap){TotalTaps=4, BitWidthIn=8, BitWidthOut=18, CoeffBitWidth=8, add_latency=1, mult_latency=2, quantization=Truncate}
      mask prompts: TotalTaps "Total Number of Taps:"; BitWidthIn "Input Bitwidth:"; BitWidthOut "Output Bitwidth:"; CoeffBitWidth "Coeff Bitwidth:"; add_latency "Add Latency"; mult_latency "Mult Latency"; quantization "Quantization Behavior"
      mask init: same as casperdemo/Complex FFT and PFB/pfb_fir/pol1_in1_last_tap
      settings: AttributesFormatString=taps=4
      mask StyleString: edit,edit,edit,edit,edit,edit,popup(Truncate|Round  (unbiased: +/- Inf)|Round  (unbiased: Even Values))
  pol1_in1_tap2 : casper_library/PFBs/tap
      link override delay/delay_bram/Constant2: equ=P=C
      link override sync_delay/Constant: equ=P=C
      link override sync_delay/Constant1: equ=P=C
      link override sync_delay/Constant2: equ=P=C
      link override sync_delay/Constant3: equ=P=C
  pol1_in1_tap3 : casper_library/PFBs/tap
      link override delay/delay_bram/Constant2: equ=P=C
      link override sync_delay/Constant: equ=P=C
      link override sync_delay/Constant1: equ=P=C
      link override sync_delay/Constant2: equ=P=C
      link override sync_delay/Constant3: equ=P=C
  pol1_in2_first_tap : Subsystem  AncestorBlock=casper_library/PFBs/first_tap  mask(first_tap){nput=1, PFBSize=5, CoeffBitWidth=8, TotalTaps=4, BitWidthIn=8, CoeffDistMem=1, WindowType=hamming, mult_latency=2, bram_latency=2, n_inputs=2, fwidth=1}
      mask prompts: nput "This is input number:"; PFBSize "Size of PFB: (2^? pnts)"; CoeffBitWidth "Bitwidth of Coefficients:"; TotalTaps "Total Number of Taps:"; BitWidthIn "Input Bitwidth:"; CoeffDistMem "Implement Coeff Gen in Distributed Memory:"; WindowType "Windowing Function:"; mult_latency "Mult Latency"; bram_latency "BRAM Latency"; n_inputs "Number of Simultaneous Inputs: (2^?)"; fwidth "Bit Width (normal=1)"
      mask init: same as casperdemo/Complex FFT and PFB/pfb_fir/pol1_in1_first_tap
      settings: AttributesFormatString=input=1, taps=4
      mask StyleString: edit,edit,edit,edit,edit,edit,popup(bartlett|barthannwin|blackman|blackmanharris|bohamwin|chebwin|flattopwin|gausswin|hamming|hann|kaiser|nuttallwin|parzenwin|rectwin|tukeywin|triang),edit,edit,edit,edit
  pol1_in2_last_tap : Subsystem  AncestorBlock=casper_library/PFBs/last_tap  mask(last_tap){TotalTaps=4, BitWidthIn=8, BitWidthOut=18, CoeffBitWidth=8, add_latency=1, mult_latency=2, quantization=Truncate}
      mask prompts: TotalTaps "Total Number of Taps:"; BitWidthIn "Input Bitwidth:"; BitWidthOut "Output Bitwidth:"; CoeffBitWidth "Coeff Bitwidth:"; add_latency "Add Latency"; mult_latency "Mult Latency"; quantization "Quantization Behavior"
      mask init: same as casperdemo/Complex FFT and PFB/pfb_fir/pol1_in1_last_tap
      settings: AttributesFormatString=taps=4
      mask StyleString: edit,edit,edit,edit,edit,edit,popup(Truncate|Round  (unbiased: +/- Inf)|Round  (unbiased: Even Values))
  pol1_in2_tap2 : casper_library/PFBs/tap
      link override delay/delay_bram/Constant2: equ=P=C
      link override sync_delay/Constant: equ=P=C
      link override sync_delay/Constant1: equ=P=C
      link override sync_delay/Constant2: equ=P=C
      link override sync_delay/Constant3: equ=P=C
  pol1_in2_tap3 : casper_library/PFBs/tap
      link override delay/delay_bram/Constant2: equ=P=C
      link override sync_delay/Constant: equ=P=C
      link override sync_delay/Constant1: equ=P=C
      link override sync_delay/Constant2: equ=P=C
      link override sync_delay/Constant3: equ=P=C
  pol1_in3_first_tap : Subsystem  AncestorBlock=casper_library/PFBs/first_tap  mask(first_tap){nput=2, PFBSize=5, CoeffBitWidth=8, TotalTaps=4, BitWidthIn=8, CoeffDistMem=1, WindowType=hamming, mult_latency=2, bram_latency=2, n_inputs=2, fwidth=1}
      mask prompts: nput "This is input number:"; PFBSize "Size of PFB: (2^? pnts)"; CoeffBitWidth "Bitwidth of Coefficients:"; TotalTaps "Total Number of Taps:"; BitWidthIn "Input Bitwidth:"; CoeffDistMem "Implement Coeff Gen in Distributed Memory:"; WindowType "Windowing Function:"; mult_latency "Mult Latency"; bram_latency "BRAM Latency"; n_inputs "Number of Simultaneous Inputs: (2^?)"; fwidth "Bit Width (normal=1)"
      mask init: same as casperdemo/Complex FFT and PFB/pfb_fir/pol1_in1_first_tap
      settings: AttributesFormatString=input=2, taps=4
      mask StyleString: edit,edit,edit,edit,edit,edit,popup(bartlett|barthannwin|blackman|blackmanharris|bohamwin|chebwin|flattopwin|gausswin|hamming|hann|kaiser|nuttallwin|parzenwin|rectwin|tukeywin|triang),edit,edit,edit,edit
  pol1_in3_last_tap : Subsystem  AncestorBlock=casper_library/PFBs/last_tap  mask(last_tap){TotalTaps=4, BitWidthIn=8, BitWidthOut=18, CoeffBitWidth=8, add_latency=1, mult_latency=2, quantization=Truncate}
      mask prompts: TotalTaps "Total Number of Taps:"; BitWidthIn "Input Bitwidth:"; BitWidthOut "Output Bitwidth:"; CoeffBitWidth "Coeff Bitwidth:"; add_latency "Add Latency"; mult_latency "Mult Latency"; quantization "Quantization Behavior"
      mask init: same as casperdemo/Complex FFT and PFB/pfb_fir/pol1_in1_last_tap
      settings: AttributesFormatString=taps=4
      mask StyleString: edit,edit,edit,edit,edit,edit,popup(Truncate|Round  (unbiased: +/- Inf)|Round  (unbiased: Even Values))
  pol1_in3_tap2 : casper_library/PFBs/tap
      link override delay/delay_bram/Constant2: equ=P=C
      link override sync_delay/Constant: equ=P=C
      link override sync_delay/Constant1: equ=P=C
      link override sync_delay/Constant2: equ=P=C
      link override sync_delay/Constant3: equ=P=C
  pol1_in3_tap3 : casper_library/PFBs/tap
      link override delay/delay_bram/Constant2: equ=P=C
      link override sync_delay/Constant: equ=P=C
      link override sync_delay/Constant1: equ=P=C
      link override sync_delay/Constant2: equ=P=C
      link override sync_delay/Constant3: equ=P=C
  pol1_in4_first_tap : Subsystem  AncestorBlock=casper_library/PFBs/first_tap  mask(first_tap){nput=3, PFBSize=5, CoeffBitWidth=8, TotalTaps=4, BitWidthIn=8, CoeffDistMem=1, WindowType=hamming, mult_latency=2, bram_latency=2, n_inputs=2, fwidth=1}
      mask prompts: nput "This is input number:"; PFBSize "Size of PFB: (2^? pnts)"; CoeffBitWidth "Bitwidth of Coefficients:"; TotalTaps "Total Number of Taps:"; BitWidthIn "Input Bitwidth:"; CoeffDistMem "Implement Coeff Gen in Distributed Memory:"; WindowType "Windowing Function:"; mult_latency "Mult Latency"; bram_latency "BRAM Latency"; n_inputs "Number of Simultaneous Inputs: (2^?)"; fwidth "Bit Width (normal=1)"
      mask init: same as casperdemo/Complex FFT and PFB/pfb_fir/pol1_in1_first_tap
      settings: AttributesFormatString=input=3, taps=4
      mask StyleString: edit,edit,edit,edit,edit,edit,popup(bartlett|barthannwin|blackman|blackmanharris|bohamwin|chebwin|flattopwin|gausswin|hamming|hann|kaiser|nuttallwin|parzenwin|rectwin|tukeywin|triang),edit,edit,edit,edit
  pol1_in4_last_tap : Subsystem  AncestorBlock=casper_library/PFBs/last_tap  mask(last_tap){TotalTaps=4, BitWidthIn=8, BitWidthOut=18, CoeffBitWidth=8, add_latency=1, mult_latency=2, quantization=Truncate}
      mask prompts: TotalTaps "Total Number of Taps:"; BitWidthIn "Input Bitwidth:"; BitWidthOut "Output Bitwidth:"; CoeffBitWidth "Coeff Bitwidth:"; add_latency "Add Latency"; mult_latency "Mult Latency"; quantization "Quantization Behavior"
      mask init: same as casperdemo/Complex FFT and PFB/pfb_fir/pol1_in1_last_tap
      settings: AttributesFormatString=taps=4
      mask StyleString: edit,edit,edit,edit,edit,edit,popup(Truncate|Round  (unbiased: +/- Inf)|Round  (unbiased: Even Values))
  pol1_in4_tap2 : casper_library/PFBs/tap
      link override delay/delay_bram/Constant2: equ=P=C
      link override sync_delay/Constant: equ=P=C
      link override sync_delay/Constant1: equ=P=C
      link override sync_delay/Constant2: equ=P=C
      link override sync_delay/Constant3: equ=P=C
  pol1_in4_tap3 : casper_library/PFBs/tap
      link override delay/delay_bram/Constant2: equ=P=C
      link override sync_delay/Constant: equ=P=C
      link override sync_delay/Constant1: equ=P=C
      link override sync_delay/Constant2: equ=P=C
      link override sync_delay/Constant3: equ=P=C
  sync_out : Outport
  pol1_out1 : Outport  Port=2
  pol1_out2 : Outport  Port=3
  pol1_out3 : Outport  Port=4
  pol1_out4 : Outport  Port=5
  wires:
  pol1_in1/1 -> pol1_in1_first_tap/1(din)
  sync/1 -> pol1_in1_first_tap/2(sync), pol1_in2_first_tap/2(sync), pol1_in3_first_tap/2(sync), pol1_in4_first_tap/2(sync)
  pol1_in1_first_tap/1(dout) -> pol1_in1_tap2/1
  pol1_in1_first_tap/2(sync_out) -> pol1_in1_tap2/2
  pol1_in1_first_tap/3(coeff_out) -> pol1_in1_tap2/3
  pol1_in1_first_tap/4(taps_out) -> pol1_in1_tap2/4
  pol1_in1_tap2/1 -> pol1_in1_tap3/1
  pol1_in1_tap2/2 -> pol1_in1_tap3/2
  pol1_in1_tap2/3 -> pol1_in1_tap3/3
  pol1_in1_tap2/4 -> pol1_in1_tap3/4
  pol1_in1_tap3/1 -> pol1_in1_last_tap/1(din)
  pol1_in1_tap3/2 -> pol1_in1_last_tap/2(sync)
  pol1_in1_tap3/3 -> pol1_in1_last_tap/3(coeff)
  pol1_in1_tap3/4 -> pol1_in1_last_tap/4(taps)
  pol1_in1_last_tap/1(dout) -> pol1_out1/1
  pol1_in1_last_tap/2(sync_out) -> sync_out/1
  pol1_in2/1 -> pol1_in2_first_tap/1(din)
  pol1_in2_first_tap/1(dout) -> pol1_in2_tap2/1
  pol1_in2_first_tap/2(sync_out) -> pol1_in2_tap2/2
  pol1_in2_first_tap/3(coeff_out) -> pol1_in2_tap2/3
  pol1_in2_first_tap/4(taps_out) -> pol1_in2_tap2/4
  pol1_in2_tap2/1 -> pol1_in2_tap3/1
  pol1_in2_tap2/2 -> pol1_in2_tap3/2
  pol1_in2_tap2/3 -> pol1_in2_tap3/3
  pol1_in2_tap2/4 -> pol1_in2_tap3/4
  pol1_in2_tap3/1 -> pol1_in2_last_tap/1(din)
  pol1_in2_tap3/2 -> pol1_in2_last_tap/2(sync)
  pol1_in2_tap3/3 -> pol1_in2_last_tap/3(coeff)
  pol1_in2_tap3/4 -> pol1_in2_last_tap/4(taps)
  pol1_in2_last_tap/1(dout) -> pol1_out2/1
  pol1_in3/1 -> pol1_in3_first_tap/1(din)
  pol1_in3_first_tap/1(dout) -> pol1_in3_tap2/1
  pol1_in3_first_tap/2(sync_out) -> pol1_in3_tap2/2
  pol1_in3_first_tap/3(coeff_out) -> pol1_in3_tap2/3
  pol1_in3_first_tap/4(taps_out) -> pol1_in3_tap2/4
  pol1_in3_tap2/1 -> pol1_in3_tap3/1
  pol1_in3_tap2/2 -> pol1_in3_tap3/2
  pol1_in3_tap2/3 -> pol1_in3_tap3/3
  pol1_in3_tap2/4 -> pol1_in3_tap3/4
  pol1_in3_tap3/1 -> pol1_in3_last_tap/1(din)
  pol1_in3_tap3/2 -> pol1_in3_last_tap/2(sync)
  pol1_in3_tap3/3 -> pol1_in3_last_tap/3(coeff)
  pol1_in3_tap3/4 -> pol1_in3_last_tap/4(taps)
  pol1_in3_last_tap/1(dout) -> pol1_out3/1
  pol1_in4/1 -> pol1_in4_first_tap/1(din)
  pol1_in4_first_tap/1(dout) -> pol1_in4_tap2/1
  pol1_in4_first_tap/2(sync_out) -> pol1_in4_tap2/2
  pol1_in4_first_tap/3(coeff_out) -> pol1_in4_tap2/3
  pol1_in4_first_tap/4(taps_out) -> pol1_in4_tap2/4
  pol1_in4_tap2/1 -> pol1_in4_tap3/1
  pol1_in4_tap2/2 -> pol1_in4_tap3/2
  pol1_in4_tap2/3 -> pol1_in4_tap3/3
  pol1_in4_tap2/4 -> pol1_in4_tap3/4
  pol1_in4_tap3/1 -> pol1_in4_last_tap/1(din)
  pol1_in4_tap3/2 -> pol1_in4_last_tap/2(sync)
  pol1_in4_tap3/3 -> pol1_in4_last_tap/3(coeff)
  pol1_in4_tap3/4 -> pol1_in4_last_tap/4(taps)
  pol1_in4_last_tap/1(dout) -> pol1_out4/1

== system casperdemo/Real FFT and Real PFB/fft_biplex_real_4x ==
  pol1 : Inport  Port=1  LatchInput=off
  pol2 : Inport  Port=2  LatchInput=off
  pol3 : Inport  Port=3  LatchInput=off
  pol4 : Inport  Port=4  LatchInput=off
  sync : Inport  Port=5  LatchInput=off
  shift : Inport  Port=6  LatchInput=off
  bi_real_unscr_4x : Subsystem  mask{FFTSize=4, bram_latency=2}
      mask prompts: FFTSize "Size of FFT (2^?):"; bram_latency "BRAM Latency"
      mask init:
      | blk = gcb;
      | 
      | set_param([blk,'/reorder'],'map', mat2str(bit_reverse(0:2^(FFTSize-1)-1, FFTSize-1)));
      | set_param([blk,'/reorder'],'bram_latency', num2str(bram_latency));
      | set_param([blk,'/reorder1'],'map', mat2str(bit_reverse(2^(FFTSize-1)-1:-1:0, FFTSize-1)));
      | set_param([blk,'/reorder1'],'bram_latency', num2str(bram_latency));
      | set_param([blk,'/reorder2'],'map', mat2str(2^(FFTSize-1)-1:-1:0));
      | set_param([blk,'/reorder2'],'bram_latency', num2str(bram_latency));
  biplex_core : Subsystem  AncestorBlock=casper_library/FFTs/biplex_core  mask(biplex_core){FFTSize=4, BitWidth=18, quantization=Truncate, overflow=Wrap, add_latency=2, mult_latency=3, bram_latency=2}
      mask prompts: FFTSize "Size of FFT: (2^? pnts)"; BitWidth "Bitwidth: (Max Efficiency at 18 bits)"; quantization "Quantization Behavior"; overflow "Overflow Behavior"; add_latency "Add Latency"; mult_latency "Mult Latency"; bram_latency "BRAM Latency"
      mask init:
      | biplex_core_init(gcb,...
      |     'FFTSize', FFTSize,...
      |     'BitWidth', BitWidth,...
      |     'quantization', quantization,...
      |     'overflow', overflow,...
      |     'add_latency', add_latency,...
      |     'mult_latency', mult_latency,...
      |     'bram_latency', bram_latency);
      settings: AttributesFormatString=FFTSize=4
      mask StyleString: edit,edit,popup(Truncate|Round  (unbiased: +/- Inf)|Round  (unbiased: Even Values)),popup(Wrap|Saturate|Error),edit,edit,edit
  ri_to_c : Subsystem
  ri_to_c1 : Subsystem
  pol1_out : Outport
  pol2_out : Outport  Port=2
  pol3_out : Outport  Port=3
  pol4_out : Outport  Port=4
  of : Outport  Port=5
  sync_out : Outport  Port=6
  wires:
  biplex_core/4(sync_out) -> bi_real_unscr_4x/3(sync)
  biplex_core/2(out2) -> bi_real_unscr_4x/2(odd)
  biplex_core/1(out1) -> bi_real_unscr_4x/1(even)
  biplex_core/3(of) -> of/1
  pol1/1 -> ri_to_c/1(re)
  ri_to_c/1(c) -> biplex_core/1(pol1)
  pol2/1 -> ri_to_c/2(im)
  pol3/1 -> ri_to_c1/1(re)
  ri_to_c1/1(c) -> biplex_core/2(pol2)
  pol4/1 -> ri_to_c1/2(im)
  sync/1 -> biplex_core/3(sync)
  shift/1 -> biplex_core/4(shift)
  bi_real_unscr_4x/1(pol1_out) -> pol1_out/1
  bi_real_unscr_4x/2(pol2_out) -> pol2_out/1
  bi_real_unscr_4x/3(pol3_out) -> pol3_out/1
  bi_real_unscr_4x/4(pol4_out) -> pol4_out/1
  bi_real_unscr_4x/5(sync_out) -> sync_out/1
